simulink model "re_written_control_system"  (R2024b)
settings: Solver=VariableStepAuto  StartTime=0.0  StopTime=4000  RelTol=1e-3
InitFcn:
  | [moter_left, moter_right, moter_bow, A ,mass, boat_dimensions, friction, inertia, wind_gain] = get_parameters(1);
  | [K, B, thuster_angle] = re_LQR();
  | rng(posixtime(datetime('now'))); % For reproducibility
  | rand_seed = rand()*1000;
values from neighbouring files (symbols this model uses):
  A = [bx/m 0 0 ... (first row only)    [calculateLQR.m]    (also in optimer.m)
  B = [sin(theta_left)*len_origen_1  , sin(theta_right)*len_origen_2  , sin(theta_3)*len_origen_3 ... (first row only)    [calculateLQR.m]    (also in optimer.m = [sin(theta_right)*len_origen_1 sin(theta_left)*len_origen_2 )
  friction = [-2, -1, -2]    [mid.m]
undefined symbols (not defined in the file or in its folder): boat_dimensions, inertia, K, mass, moter_bow, moter_left, moter_right, thuster_angle, wind_gain
libraries: simulink_extras x3
settings Model: Creator=klyx  LastModifiedBy=klyx

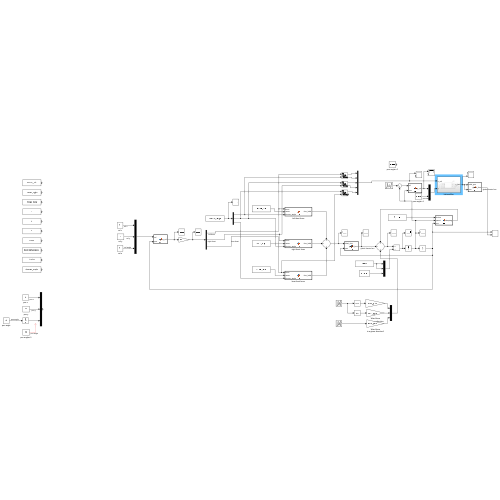
[thumbnail: Simulink's stored preview of the top-level diagram]
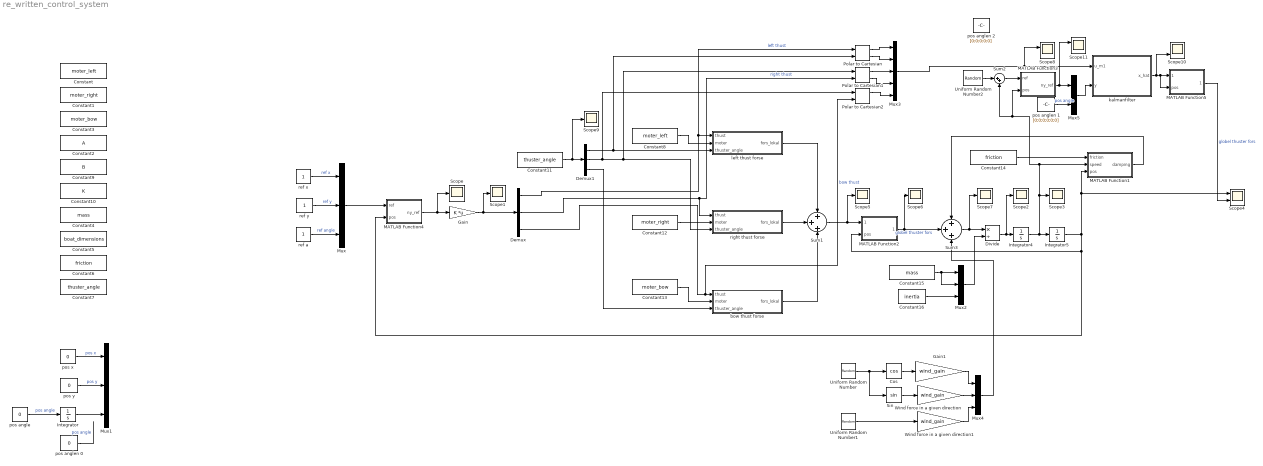
== system re_written_control_system ==
  Constant : Constant  Value=moter_left
  Constant1 : Constant  Value=moter_right
  Constant10 : Constant  Value=K
  Constant11 : Constant  Value=thuster_angle
  Constant12 : Constant  Value=moter_right
  Constant13 : Constant  Value=moter_bow
  Constant14 : Constant  Value=friction
  Constant15 : Constant  Value=mass
  Constant16 : Constant  Value=inertia
  Constant2 : Constant  Value=A
  Constant3 : Constant  Value=moter_bow
  Constant4 : Constant  Value=mass
  Constant5 : Constant  Value=boat_dimensions
  Constant6 : Constant  Value=friction
  Constant7 : Constant  Value=thuster_angle
  Constant8 : Constant  Value=moter_left
  Constant9 : Constant  Value=B
  Cos : Trigonometry  Operator=cos
  Demux : Demux  Outputs=3
  Demux1 : Demux  Outputs=3
  Divide : Product  Inputs=*/
  Gain : Gain  Gain=K  Multiplication=Matrix(K*u)
  Gain1 : Gain  Gain=wind_gain
  Integrator : Integrator
  Integrator4 : Integrator  InitialCondition=[0; 0; 0]
  Integrator5 : Integrator  InitialCondition=[0; 0; 0]
  MATLAB Function1 : MATLAB Function  TreatAsAtomicUnit=on
  MATLAB Function2 : MATLAB Function  TreatAsAtomicUnit=on
  MATLAB Function3 : MATLAB Function  TreatAsAtomicUnit=on
  MATLAB Function4 : MATLAB Function  TreatAsAtomicUnit=on
  MATLAB Function5 : MATLAB Function  TreatAsAtomicUnit=on
  Mux{,1..2,4} (4 alike) : Mux  Inputs=3
  Mux3 : Mux  Inputs=5
  Mux5 : Mux  Inputs=2
  Polar to Cartesian : simulink_extras/Transformations/Polar to Cartesian
  Polar to Cartesian1 : simulink_extras/Transformations/Polar to Cartesian
  Polar to Cartesian2 : simulink_extras/Transformations/Polar to Cartesian
  Scope{,1..3,5..7,9} (8 alike) : Scope
  Scope{4,8,10..11} (4 alike) : Scope  NumInputPorts=2
  Sin : Trigonometry
  Sum1 : Sum  Inputs=+++
  Sum2 : Sum  Inputs=|++
  Sum3 : Sum  Inputs=+++
  Uniform Random Number : UniformRandomNumber  Minimum=0  Maximum=6.28  Seed=rand_seed  SampleTime=1
  Uniform Random Number1 : UniformRandomNumber  Minimum=-6.28  Maximum=6.28  Seed=rand_seed+1  SampleTime=1
  Uniform Random Number2 : UniformRandomNumber  Minimum=-2  Maximum=2  Seed=1  SampleTime=1
  Wind force in a given direction : Gain  Gain=wind_gain
  Wind force in a given direction1 : Gain  Gain=wind_gain
  bow thust forse : MATLAB Function  TreatAsAtomicUnit=on
  kalmanfilter : Subsystem
  left thust forse : MATLAB Function  TreatAsAtomicUnit=on
  pos angle : Constant  Value=0
  pos anglen 0 : Constant  Value=0
  pos anglen 1 : Constant  Value=[0;0;0;0;0;0]
  pos anglen 2 : Constant  Value=[0;0;0;0;0]
  pos x : Constant  Value=0
  pos y : Constant  Value=0
  ref a : Constant
  ref x : Constant
  ref y : Constant
  right thust forse : MATLAB Function  TreatAsAtomicUnit=on
  wires:
  ref x/1 -> Mux/1  "ref x"
  ref y/1 -> Mux/2  "ref y"
  ref a/1 -> Mux/3  "ref angle"
  pos y/1 -> Mux1/2  "pos y"
  pos x/1 -> Mux1/1  "pos x"
  pos angle/1 -> Integrator/1  "pos angle"
  MATLAB Function4/1(ny_ref) -> Scope/1, Gain/1
  pos anglen 0/1 -> ?  "pos angle"
  Integrator/1 -> Mux1/3
  Gain/1 -> Scope1/1, Demux/1
  Demux/1 -> Polar to Cartesian/1, left thust forse/1(thust)  "left thust"
  Demux/3 -> Polar to Cartesian2/2, bow thust forse/1(thust)  "bow thust"
  Constant8/1 -> left thust forse/2(moter)
  Constant11/1 -> Scope9/1, Demux1/1
  Demux1/1 -> left thust forse/3(thuster_angle), Polar to Cartesian/2
  Constant13/1 -> bow thust forse/2(moter)
  Demux/2 -> Polar to Cartesian1/2, right thust forse/1(thust)  "right thust"
  Demux1/3 -> bow thust forse/3(thuster_angle)
  Constant12/1 -> right thust forse/2(moter)
  Integrator5/1 -> Scope4/1, MATLAB Function1/3(pos), MATLAB Function2/2(pos), MATLAB Function4/2(pos)
  Constant15/1 -> Mux2/2, Mux2/1
  Sum1/1 -> MATLAB Function2/1(lokal_fors), Scope5/1
  Integrator4/1 -> Integrator5/1, Scope3/1, MATLAB Function3/2(pos), Sum2/2, MATLAB Function1/2(speed)
  Mux2/1 -> Divide/2
  Divide/1 -> Scope2/1, Integrator4/1
  Constant16/1 -> Mux2/3
  MATLAB Function1/1(damping) -> Sum3/1
  Sum3/1 -> Scope7/1, Divide/1
  Constant14/1 -> MATLAB Function1/1(friction)
  MATLAB Function2/1(globel_fors) -> Scope6/1, Sum3/2  "globel thuster fors"
  Mux/1 -> MATLAB Function4/1(ref)
  Uniform Random Number/1 -> Sin/1, Cos/1
  Cos/1 -> Gain1/1
  Sin/1 -> Wind force in a given direction/1
  Uniform Random Number1/1 -> Wind force in a given direction1/1
  Gain1/1 -> Mux4/1
  Wind force in a given direction/1 -> Mux4/2
  Wind force in a given direction1/1 -> Mux4/3
  Mux4/1 -> Sum3/3
  right thust forse/1(fors_lokal) -> Sum1/2
  left thust forse/1(fors_lokal) -> Sum1/1
  bow thust forse/1(fors_lokal) -> Sum1/3
  Sum2/1 -> MATLAB Function3/1(ref)
  Uniform Random Number2/1 -> Sum2/1
  Demux1/2 -> Polar to Cartesian2/1, Polar to Cartesian1/1, right thust forse/3(thuster_angle)
  Polar to Cartesian/1 -> Mux3/1
  Polar to Cartesian/2 -> Mux3/2
  Polar to Cartesian1/1 -> Mux3/3
  Polar to Cartesian1/2 -> Mux3/4
  kalmanfilter/1(x_hat) -> Scope10/2, MATLAB Function5/2(pos), MATLAB Function5/1(lokal_pos)
  pos anglen 1/1 -> Mux5/2  "pos angle"
  Mux5/1 -> kalmanfilter/2(y)
  Polar to Cartesian2/1 -> Mux3/5
  MATLAB Function3/1(ny_ref) -> Scope11/1, Mux5/1
  Mux3/1 -> Scope8/1, kalmanfilter/1(u_m1)
  MATLAB Function5/1(globel_fors) -> Scope4/2  "globel thuster fors"

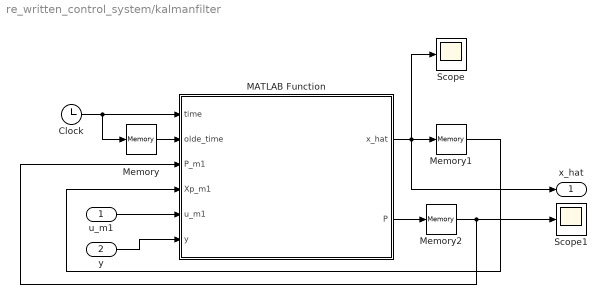
== system re_written_control_system/kalmanfilter ==
  u_m1 : Inport
  y : Inport  Port=2
  Clock : Clock
  MATLAB Function : MATLAB Function  TreatAsAtomicUnit=on
  Memory : Memory
  Memory1 : Memory  InitialCondition=[0;0;0;1;1;1;0;0;0]
  Memory2 : Memory  InitialCondition=eye(9) * 1e-3;
  Scope : Scope
  Scope1 : Scope
  x_hat : Outport
  wires:
  Memory/1 -> MATLAB Function/2(olde_time)
  Memory2/1 -> Scope1/1, MATLAB Function/3(P_m1)
  MATLAB Function/2(P) -> Memory2/1
  Memory1/1 -> MATLAB Function/4(Xp_m1)
  y/1 -> MATLAB Function/6(y)
  MATLAB Function/1(x_hat) -> Scope/1, x_hat/1, Memory1/1
  Clock/1 -> MATLAB Function/1(time), Memory/1
  u_m1/1 -> MATLAB Function/5(u_m1)

== matlab function re_written_control_system/MATLAB Function1 ==
  data: friction input; damping output; speed input; pos input
function damping = fcn(friction, speed, pos)

firk = [friction(1) 0           0           ;
        0           friction(2) 0           ;
        0           0           friction(3)];

glo_to_lok = [cos(-pos(3)) -sin(-pos(3)) 0 ;
              sin(-pos(3)) cos(-pos(3))  0 ;
              0           0              1];

%s = speed
%rotl = inv(glo_to_lok)*firk*glo_to_lok;
damping = inv(glo_to_lok)*firk*glo_to_lok*speed;

== matlab function re_written_control_system/MATLAB Function4 ==
  data: ref input; ny_ref output; pos input
function ny_ref = fcn(ref ,pos)

xy_pos = [0 0 ref(1);
          0 0 ref(2);
          0 0 1];

glo_to_lok = [cos(pos(3)) -sin(pos(3)) pos(1);
              sin(pos(3)) cos(pos(3))  pos(2);
              0           0            1];

lok_ref = inv(glo_to_lok)*xy_pos;
ny_ref  = [-lok_ref(1,3); -lok_ref(2,3); ref(3)- pos(3)];

%lok_ref = inv(glo_to_lok)*xy_pos;
%ny_ref  = [lok_ref(1,3) - pos(1); lok_ref(2,3) - pos(2); ref(3)- pos(3)];

== matlab function re_written_control_system/bow thust forse ==
  data: thust input; fors_lokal output; moter input; thuster_angle input
function fors_lokal  = fcn(thust, moter, thuster_angle)
%this is the in the boat local frame
Fx     = cos(thuster_angle)*thust;
Fy     = sin(thuster_angle)*thust;
torque = sin(moter(3)+thuster_angle)*moter(4)*thust;
fors_lokal = [Fx, Fy, torque];

== matlab function re_written_control_system/left thust forse ==
  data: thust input; fors_lokal output; moter input; thuster_angle input
function fors_lokal = fcn(thust, moter, thuster_angle)
%this is the in the boat local frame
Fx     = cos(thuster_angle)*thust;
Fy     = sin(thuster_angle)*thust;
torque = sin(moter(3)+thuster_angle)*moter(4)*thust;
fors_lokal = [Fx, Fy, torque];

== matlab function re_written_control_system/MATLAB Function2 ==
  data: lokal_fors input; globel_fors output; pos input
function globel_fors = fcn(lokal_fors ,pos)

xy_pos = [lokal_fors(1);lokal_fors(2)];

glo_to_lok = [cos(pos(3)) -sin(pos(3));
              sin(pos(3)) cos(pos(3))];

gb_xy_fors = inv(glo_to_lok)*xy_pos;

globel_fors  = [gb_xy_fors(1);gb_xy_fors(2); lokal_fors(3)];

== matlab function re_written_control_system/right thust forse ==
  data: thust input; fors_lokal output; moter input; thuster_angle input
function fors_lokal  = fcn(thust, moter, thuster_angle)
%this is the in the boat local frame
Fx     = cos(thuster_angle)*thust;
Fy     = sin(thuster_angle)*thust;
torque = sin(moter(3)+thuster_angle)*moter(4)*thust;
fors_lokal = [Fx, Fy, torque];

== matlab function re_written_control_system/kalmanfilter/MATLAB Function ==
  data: time input; x_hat output; olde_time input; P_m1 input; Xp_m1 input; u_m1 input; y input; P output
function [x_hat, P] = extended_kalman_filter_sim(time, olde_time, P_m1, Xp_m1, u_m1, y)
    % Time step
    td = time - olde_time;
    length_x = 2.74;
    length_y = 5.32;
    c = -1;
    moter_left  = [-length_x/2, -length_y/2+c, 0, 0];
    moter_right = [ length_x/2, -length_y/2+c, 0, 0];
    moter_bow   = [ 0,           length_y+c  , 0, 0];

    m = 1500; % Mass of the boat
    I = (length_y^2+length_x^2)*m*1/12;
    % Known parameters
    bx = -0;
    by = -0;
    bt = -0;
    t1x = moter_left(1);
    y1  = moter_left(2);
    %moter 2
    t2x = moter_right(1);
    y2  = moter_right(2);
    %moter 3
    t3x = moter_bow(1);
    y3  = moter_bow(2);


    % Noise covariances
    Q_m1 = diag([1e-5, 1e-5, 1e-5, 1e-5, 1e-5, 1e-5, 1e-4, 1e-4, 1e-4]); % Smaller process noise for bc
    R    = diag([1e-2, 1e-2, 1e-2, 1e-3, 1e-3, 1e-3, 1e-1, 1e-1, 1e-1]);    % Smaller measurement noise for velocity

    % State transition model
    A = [0 0 0 1 0 0 0 0 0; 0 0 0 0 1 0 0 0 0; 0 0 0 0 0 1 0 0 0; 0 0 0 bx/m-Xp_m1(7)/m 0 0 0 0 0; 0 0 0 0 by/m-Xp_m1(8)/m 0 0 0 0; 0 0 0 0 0 bt/I-Xp_m1(9)/I 0 0 0; 0 0 0 0 0 0 0 0 0; 0 0 0 0 0 0 0 0 0; 0 0 0 0 0 0 0 0 0];
    c = diag([1; 1; 1; 0; 0; 0; 0; 0; 0]);
    f = @(xp_m1, u_m1) xp_m1+[0 0 0 1 0 0 0 0 0;
                              0 0 0 0 1 0 0 0 0;
                              0 0 0 0 0 1 0 0 0;
                              0 0 0 bx/m-xp_m1(7)/m 0 0 0 0 0; 
                              0 0 0 0 by/m-xp_m1(8)/m 0 0 0 0;
                              0 0 0 0 0 bt/I-xp_m1(9)/I 0 0 0;
                              0 0 0 0 0 0 0 0 0;
                              0 0 0 0 0 0 0 0 0;
                              0 0 0 0 0 0 0 0 0]*xp_m1*td + [0,0,0,0,0;
                                                             0,0,0,0,0;
                                                             0,0,0,0,0;
                                                             1,0,1,0,1;
                                                             0,1,0,1,0;
                                                             -y1/m, t1x/m, -y2/m, t2x/m, -y3/m;
                                                             0,0,0,0,0;
                                                             0,0,0,0,0;
                                                             0,0,0,0,0]*td*u_m1;
    % syms x1 x2 x3 x4 x5 x6 x7 x8 x9 bx by bt m I y1 y2 y3 t1x t2x td
    % xp_m1 = [x1; x2; x3; x4; x5; x6; x7; x8; x9]
    % f = ...
    % jacobian(f(xp_m1, [1;1;1;1;1]),xp_m1)
    F_m1 = @(x) [1, 0, 0,                   td,                    0,                    0,            0,            0,            0;
                 0, 1, 0,                    0,                   td,                    0,            0,            0,            0;
                 0, 0, 1,                    0,                    0,                   td,            0,            0,            0;
                 0, 0, 0, td*(bx/m-x(7)/m) + 1,                    0,                    0, -(td*x(4))/m,            0,            0;
                 0, 0, 0,                    0, td*(by/m-x(8)/m) + 1,                    0,            0, -(td*x(5))/m,            0;
                 0, 0, 0,                    0,                    0, td*(bt/I-x(9)/I) + 1,            0,            0, -(td*x(6))/I;
                 0, 0, 0,                    0,                    0,                    0,            1,            0,            0;
                 0, 0, 0,                    0,                    0,                    0,            0,            1,            0;
                 0, 0, 0,                    0,                    0,                    0,            0,            0,            1];
    % Measurement model
    h = @(xp_m1) [xp_m1(1); xp_m1(2); xp_m1(3); 0; 0; 0; 0; 0; 0];
    L_m1 = @(w) eye(9);
    H_f = @(Xp_m1) diag([1; 1; 1; 0; 0; 0; 0; 0; 0]);% C matrix
    M_f = @(Xp_m1) eye(9);

    H = H_f(Xp_m1);
    M = M_f(Xp_m1);
    I = eye(9);

    Pm = F_m1(Xp_m1)*P_m1*F_m1(Xp_m1)' + L_m1(Xp_m1)*Q_m1*L_m1(Xp_m1)';
    Xm = f(Xp_m1,u_m1);
    
    %rank(obsv(F_m1(Xp_m1),H))
    %cond(obsv(F_m1(Xp_m1),H));

    K = Pm * H' / (H * Pm * H' + M * R * M');
    Xp = Xm + K*(y-h(Xp_m1));
    Pp = (I - K*H)*Pm*(I - K*H)' + K*R*K';
    P = Pp;
    x_hat = Xp;   % Updated covariance
end

== matlab function re_written_control_system/MATLAB Function3 ==
  data: ref input; ny_ref output; pos input
function ny_ref = fcn(ref ,pos)

xy_pos = [0 0 ref(1);
          0 0 ref(2);
          0 0 1];

glo_to_lok = [cos(pos(3)) -sin(pos(3)) 0;
              sin(pos(3)) cos(pos(3))  0;
              0           0            1];

lok_ref = inv(glo_to_lok)*xy_pos;
ny_ref  = [lok_ref(1,3); lok_ref(2,3); pos(3)];

== matlab function re_written_control_system/MATLAB Function5 ==
  data: lokal_pos input; globel_fors output; pos input
function globel_fors = fcn(lokal_pos ,pos)

glo_to_lok =eye(9) + [cos(pos(3)) -sin(pos(3)) 0 0 0 0 0 0 0;
                      sin(pos(3))  cos(pos(3)) 0 0 0 0 0 0 0
                      0            0           1 0 0 0 0 0 0
                      0            0           0 cos(pos(3)) -sin(pos(3)) 0 0 0 0
                      0            0           0 sin(pos(3))  cos(pos(3)) 0 0 0 0
                      0            0           0           0            0 1 0 0 0
                      0            0           0           0            0 0 1 0 0
                      0            0           0           0            0 0 0 1 0
                      0            0           0           0            0 0 0 0 1];

gb_xy_fors = inv(glo_to_lok)*lokal_pos;

globel_fors  = [gb_xy_fors(1);gb_xy_fors(2); gb_xy_fors(3)];
